simulink model "Leda"  (Simulink 7.9)
settings: Solver=ode45  StartTime=0.0  StopTime=inf  RelTol=1e-3
undefined symbols (not defined in the file or in its folder): get
libraries: dspsnks4 x2, simulink x1, dspsrcs4 x1
settings Model: Creator=agus  LastModifiedBy=Pablo
settings CodeAppCC: CustomSymbolStrType=$N$R$M_T

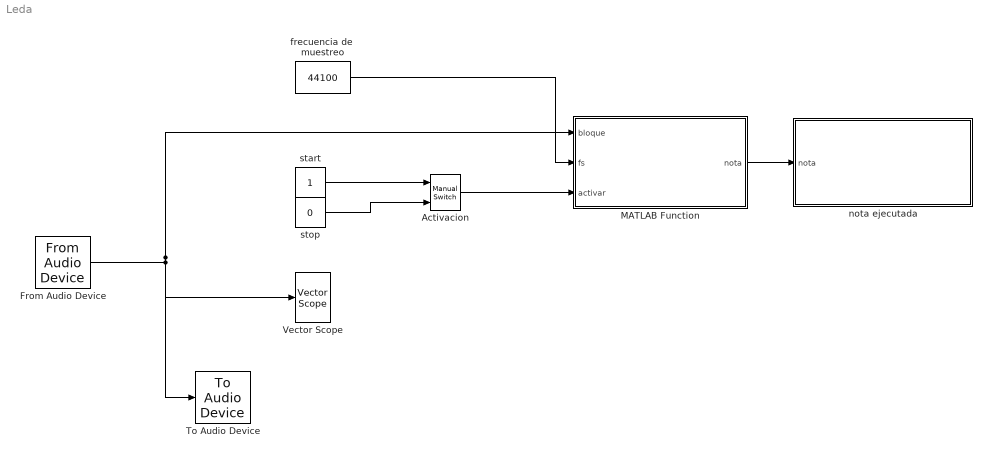
== system Leda ==
  Activacion : simulink/Signal Routing/Manual Switch  sw=1  action=0  varsize=off
  From Audio Device : dspsrcs4/From Audio Device  deviceName=ASIO4ALL v2  numChannels=1  sampleRate=44100  deviceDatatype=16-bit integer  autoBufferSize=off  bufferSize=256  queueDuration=1.0  frameSize=256  outputDatatype=double
  MATLAB Function : MATLAB Function  TreatAsAtomicUnit=on
  To Audio Device : dspsnks4/To Audio Device  deviceName=ASIO4ALL v2  inheritSampleRate=on  sampleRate=44100  deviceDatatype=Determine from input data type  autoBufferSize=off  bufferSize=256  queueDuration=1.0
  Vector Scope : dspsnks4/Vector Scope  ScopeProperties=on  Domain=Time  HorizSpan=1  DisplayProperties=off  AxisGrid=on  Memory=off  FrameNumber=on  AxisLegend=off  AxisZoom=off  OpenScopeAtSimStart=on  OpenScopeImmediately=off  FigPos=get(0,'defaultfigureposition')  AxisProperties=off  XUnits=Hertz  XRange=[0...Fs/2]  InheritXIncr=on  XIncr=1  XLabel=Time  XLimit=Auto  XMin=0  XMax=1  XStart=0  YUnits=dB  YLabel=Amplitude  LineProperties=off  XAxisParamsVer=6.9
      settings: YMin=-10  YMax=10
  frecuencia de  muestreo : Constant  Value=44100
  nota ejecutada : MATLAB Function  TreatAsAtomicUnit=on
  start : Constant
  stop : Constant  Value=0
  wires:
  From Audio Device/1 -> To Audio Device/1, MATLAB Function/1(bloque), Vector Scope/1
  MATLAB Function/1(nota) -> nota ejecutada/1(nota)
  start/1 -> Activacion/1
  stop/1 -> Activacion/2
  Activacion/1 -> MATLAB Function/3(activar)
  frecuencia de  muestreo/1 -> MATLAB Function/2(fs)

== matlab function MATLAB Function ==
  data: bloque input double; fs input double; activar input double; nota output double
function nota =Bloque_Detector(bloque, fs, activar)

    persistent f_dur;
    persistent f_detec;
            
    frec_Ffund = ' ';
    nota = 4;

    if activar
        
        %% ******** INICIALIZACION ********** %

            % clc;
            % clear all;
            % close all;

            % Asignacion de valores a las variables intervinientes en funcion de
            % las caracteristicas del archivo

            % window_len es cantidad de muestras a analizar (bloque)
            % salto es el desplazamiento respecto a la primer muestra del bloque
            % analizado con anterioridad, a partir del cual se comforma el segundo
            % bloque de analisis
            dur_len = 1024;  
            detec_len = 2048;  
            salto = 256;      


        %% ******** DURACION ********** %
            
            
            if isempty(f_dur)
                f_dur = 0;
                f_detec = 0;
            end
            
            nota = dur_prueba_simulink(bloque, dur_len, salto, fs);
            
            if nota == 2
                f_dur = f_dur+1;
            elseif nota == 0
                f_dur = 0;
            end
                

        %% ********* DETECTOR ************ %
        
            in = 0;
            
            if f_dur == 4
                if f_detec == 0
                    in = bloque;
                else
                    in = [in ; bloque];
                end
                f_detec = f_detec+1;
                
                %if f_detec == detec_len/salto
                if length(in) == 2048
                    [~,nota]=FindPitch_simulink(in', 2048,fs,80);   % llamado a deteccion de tono (carpeta funciones\Pitch Detection)
                end
                
            end


    end


end

== matlab function nota ejecutada ==
  data: nota input double
function pentagrama(nota)

eml.extrinsic('num2str');
eml.extrinsic('imread');


persistent pent;

if isempty(pent)
    pent = zeros(381,381,3,76); 
    for i = 4:76

        pent(:,:,:,i) = imread([num2str(i) '.jpg']);
        
    end
end

%% PENTAGRAMA entrega la imagen de la nota en un pentagrama
if nota < 4
    nota = 4;
end
if nota > 76
    nota =76;
end

eml.extrinsic('imshow'); % para lograr compatibilidad con simulink
% leo a traves de I=imread('im.jpg')

% muestro la imagen que corresponde en funcion de la nota que debo
% representar traves de imshow(I)

imshow(pent(:,:,:,nota));

end
